simulink library "SDC_decoder_lib"  (Simulink 7.4)
settings: Solver=ode45  StartTime=0.0  StopTime=10.0  RelTol=1e-3
values from neighbouring files (symbols this model uses):
  sPunc_pat = struct( 'Rp16' ,{[1 1 1 1 1 1]' 1 6}, 'Rp14' ,{[1 1 1 1 0 0]' 1 4}, 'Rp310',{[1 1 1 1 0 0 1 1 1 0 0 0 1 1 1 0 0 0]' 3 10}, 'Rp13' ,{[1 1 1 0 0 0]' 1 3}, 'Rp411',{[1 1 1 0 0 0 1 1 1 0 0 0 1 1 1 0 0 0 1 1 0 0 0 0]' 4 11}, 'Rp25',{[1 1 1 0 0 0 1 1 0 0 0]' 2 5}, 'Rp12',{[1 1 0 0 0 0]' 1 2}, 'Rp47' ,{[1 1 0 0 0 0 1 0 1 0 0 0 1 1 0 0 0 0 1 0 0 0 0 0]' 4 7}, 'Rp35' ,{[1 1 0 0 0 0 1 0 0 0 0 0 1 1 0 0 0 0] ...(+501 chars)    [conv_and_puncturing.m]
undefined symbols (not defined in the file or in its folder): sdc
libraries: dspmtrx3 x9, commsequence2 x6, commutil2 x3, commcnvcod2 x3, commblkintrlv2 x3, dspbuff3 x3, commdigbbndam3 x2, SDC_decoder_lib x1
settings Model: Creator=Kevin  LastModifiedBy=Kevin

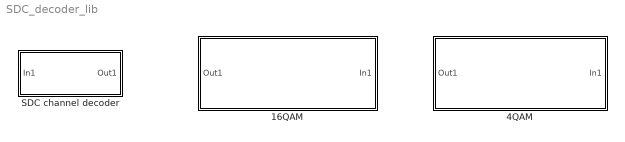
== system SDC_decoder_lib ==
  16QAM : Subsystem
  4QAM : Subsystem
  SDC channel decoder : Subsystem  BlockChoice=16QAM
      settings: TemplateBlock=self  MemberBlocks=16QAM,4QAM

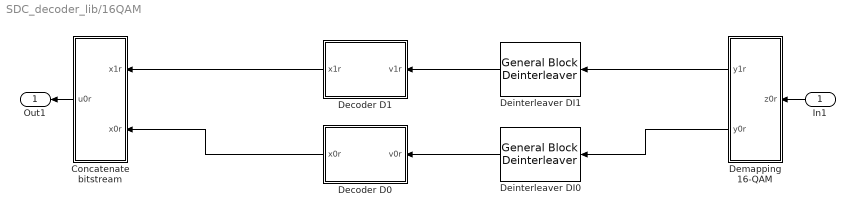
== system SDC_decoder_lib/16QAM ==
  In1 : Inport
  Concatenate bitstream : Subsystem
  Decoder D0 : Subsystem
  Decoder D1 : Subsystem
  Deinterleaver DI0 : commblkintrlv2/General Block Deinterleaver  elements=sdc.interleave_P0
  Deinterleaver DI1 : commblkintrlv2/General Block Deinterleaver  elements=sdc.interleave_P1
  Demapping 16-QAM : Subsystem
  Out1 : Outport
  wires:
  Deinterleaver DI0/1 -> Decoder D0/1(v0r)
  Deinterleaver DI1/1 -> Decoder D1/1(v1r)
  Decoder D0/1(x0r) -> Concatenate bitstream/2(x0r)
  Decoder D1/1(x1r) -> Concatenate bitstream/1(x1r)
  Demapping 16-QAM/2(y0r) -> Deinterleaver DI0/1
  Demapping 16-QAM/1(y1r) -> Deinterleaver DI1/1
  Concatenate bitstream/1(u0r) -> Out1/1
  In1/1 -> Demapping 16-QAM/1(z0r)

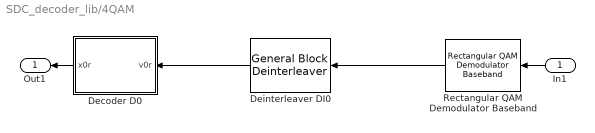
== system SDC_decoder_lib/4QAM ==
  In1 : Inport
  Decoder D0 : Subsystem
  Deinterleaver DI0 : commblkintrlv2/General Block Deinterleaver  elements=sdc.interleave_P0
  Rectangular QAM Demodulator Baseband : commdigbbndam3/Rectangular QAM Demodulator Baseband  DialogController=commDDGCreate  DialogControllerArgs=DataTag4  M=SDC_QAM  PowType=Min. distance between symbols  MinDist=sdc.qam_norm  AvgPow=1  PeakPow=1  Ph=0  Dec=User-defined  Mapping=sdc.qam_map  OutType=Bit  DecType=Hard decision  VarSource=Dialog  Variance=1  outDtype1=Inherit via internal rule  outDtype2=Inherit via internal rule  derotateFactorWordLen=16  denormFactorWordLen=16  prodOutWordLen=32  prodOutRoundingMode=Floor  prodOutOverflowMode=Wrap  sumWordLen=32
  Out1 : Outport
  wires:
  Rectangular QAM Demodulator Baseband/1 -> Deinterleaver DI0/1
  Deinterleaver DI0/1 -> Decoder D0/1(v0r)
  Decoder D0/1(x0r) -> Out1/1
  In1/1 -> Rectangular QAM Demodulator Baseband/1

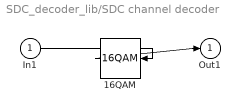
== system SDC_decoder_lib/SDC channel decoder ==
  In1 : Inport
  16QAM : SDC_decoder_lib/16QAM  SystemSampleTime=-1
  Out1 : Outport
  wires:
  In1/1 -> 16QAM/1
  16QAM/1 -> Out1/1

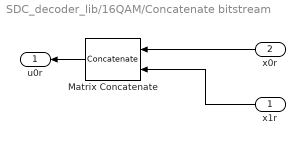
== system SDC_decoder_lib/16QAM/Concatenate bitstream ==
  x1r : Inport
  x0r : Inport  Port=2
  Matrix Concatenate : Concatenate  Mode=Multidimensional array
  u0r : Outport
  wires:
  Matrix Concatenate/1 -> u0r/1
  x0r/1 -> Matrix Concatenate/1
  x1r/1 -> Matrix Concatenate/2

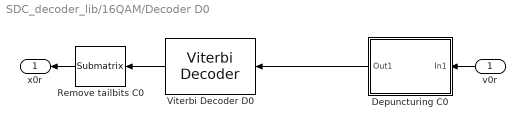
== system SDC_decoder_lib/16QAM/Decoder D0 ==
  v0r : Inport
  Depuncturing C0 : Subsystem
  Remove tailbits C0 : dspmtrx3/Submatrix  RowSpan=Range of rows  RowStartMode=First  RowStartIndex=1  RowEndMode=Offset from last  RowEndIndex=6  ColSpan=All columns  ColStartMode=First  ColStartIndex=1  ColEndMode=Last  ColEndIndex=1
  Viterbi Decoder D0 : commcnvcod2/Viterbi Decoder  DialogController=commDDGCreate  DialogControllerArgs=DataTag0  trellis=conv_poly  isPunctured=off  punctureVector=sPunc_pat(1).Rp13  erasures=off  dectype=Unquantized  runSigValErrCheck=on  nsdecb=3  smWordLength=16  tbdepth=34  opmode=Terminated  reset=off  outDataType=Inherit via internal rule
  x0r : Outport
  wires:
  Remove tailbits C0/1 -> x0r/1
  v0r/1 -> Depuncturing C0/1(In1)
  Depuncturing C0/1(Out1) -> Viterbi Decoder D0/1
  Viterbi Decoder D0/1 -> Remove tailbits C0/1

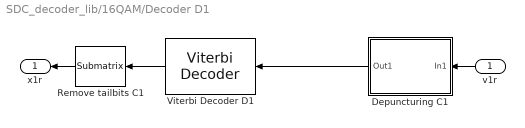
== system SDC_decoder_lib/16QAM/Decoder D1 ==
  v1r : Inport
  Depuncturing C1 : Subsystem
  Remove tailbits C1 : dspmtrx3/Submatrix  RowSpan=Range of rows  RowStartMode=First  RowStartIndex=1  RowEndMode=Offset from last  RowEndIndex=6  ColSpan=All columns  ColStartMode=First  ColStartIndex=1  ColEndMode=Last  ColEndIndex=1
  Viterbi Decoder D1 : commcnvcod2/Viterbi Decoder  DialogController=commDDGCreate  DialogControllerArgs=DataTag1  trellis=conv_poly  isPunctured=off  punctureVector=sPunc_pat(1).Rp23  erasures=off  dectype=Unquantized  runSigValErrCheck=on  nsdecb=3  smWordLength=16  tbdepth=34  opmode=Terminated  reset=off  outDataType=Inherit via internal rule
  x1r : Outport
  wires:
  Remove tailbits C1/1 -> x1r/1
  v1r/1 -> Depuncturing C1/1(In1)
  Depuncturing C1/1(Out1) -> Viterbi Decoder D1/1
  Viterbi Decoder D1/1 -> Remove tailbits C1/1

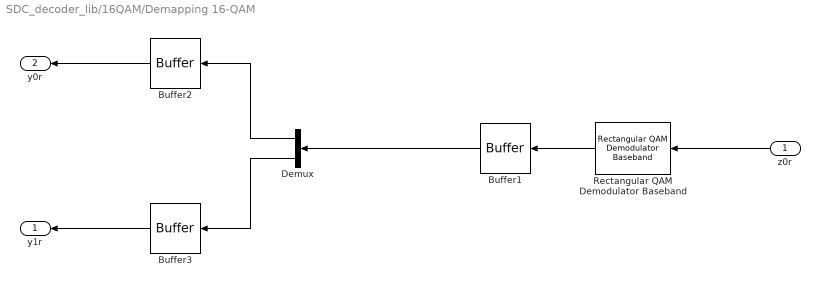
== system SDC_decoder_lib/16QAM/Demapping 16-QAM ==
  z0r : Inport
  Buffer1 : dspbuff3/Buffer  N=2  V=0  ic=0
  Buffer2 : dspbuff3/Buffer  N=2*sdc.NmbQAMcells  V=0  ic=0
  Buffer3 : dspbuff3/Buffer  N=2*sdc.NmbQAMcells  V=0  ic=0
  Demux : Demux  Outputs=2
  Rectangular QAM Demodulator Baseband : commdigbbndam3/Rectangular QAM Demodulator Baseband  DialogController=commDDGCreate  DialogControllerArgs=DataTag2  M=SDC_QAM  PowType=Min. distance between symbols  MinDist=sdc.qam_norm  AvgPow=1  PeakPow=1  Ph=0  Dec=User-defined  Mapping=sdc.qam_map  OutType=Bit  DecType=Hard decision  VarSource=Dialog  Variance=1  outDtype1=Inherit via internal rule  outDtype2=Inherit via internal rule  derotateFactorWordLen=16  denormFactorWordLen=16  prodOutWordLen=32  prodOutRoundingMode=Floor  prodOutOverflowMode=Wrap  sumWordLen=32
  y1r : Outport
  y0r : Outport  Port=2
  wires:
  z0r/1 -> Rectangular QAM Demodulator Baseband/1
  Rectangular QAM Demodulator Baseband/1 -> Buffer1/1
  Demux/2 -> Buffer3/1
  Demux/1 -> Buffer2/1
  Buffer2/1 -> y0r/1
  Buffer3/1 -> y1r/1
  Buffer1/1 -> Demux/1

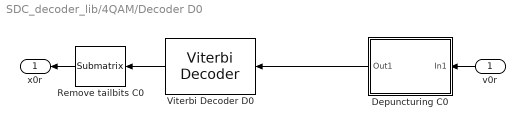
== system SDC_decoder_lib/4QAM/Decoder D0 ==
  v0r : Inport
  Depuncturing C0 : Subsystem
  Remove tailbits C0 : dspmtrx3/Submatrix  RowSpan=Range of rows  RowStartMode=First  RowStartIndex=1  RowEndMode=Offset from last  RowEndIndex=6  ColSpan=All columns  ColStartMode=First  ColStartIndex=1  ColEndMode=Last  ColEndIndex=1
  Viterbi Decoder D0 : commcnvcod2/Viterbi Decoder  DialogController=commDDGCreate  DialogControllerArgs=DataTag3  trellis=conv_poly  isPunctured=off  punctureVector=sPunc_pat(1).Rp13  erasures=off  dectype=Unquantized  runSigValErrCheck=on  nsdecb=3  smWordLength=16  tbdepth=34  opmode=Terminated  reset=off  outDataType=Inherit via internal rule
  x0r : Outport
  wires:
  Remove tailbits C0/1 -> x0r/1
  v0r/1 -> Depuncturing C0/1(In1)
  Depuncturing C0/1(Out1) -> Viterbi Decoder D0/1
  Viterbi Decoder D0/1 -> Remove tailbits C0/1

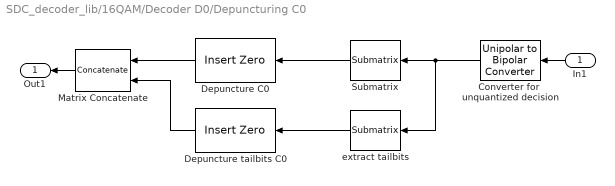
== system SDC_decoder_lib/16QAM/Decoder D0/Depuncturing C0 ==
  In1 : Inport
  Converter for  unquantized decision : commutil2/Unipolar to Bipolar Converter  SystemSampleTime=-1  M=2  polarity=Negative  dataType=Inherit via internal rule
  Depuncture C0 : commsequence2/Insert Zero  insertZeroVector=sdc.punc_pat0
  Depuncture tailbits C0 : commsequence2/Insert Zero  insertZeroVector=sdc.punc_tail0
  Matrix Concatenate : Concatenate  Mode=Multidimensional array
  Submatrix : dspmtrx3/Submatrix  RowSpan=Range of rows  RowStartMode=First  RowStartIndex=1  RowEndMode=Offset from last  RowEndIndex=sdc.ind_tail0  ColSpan=All columns  ColStartMode=First  ColStartIndex=1  ColEndMode=Last  ColEndIndex=1
  extract tailbits : dspmtrx3/Submatrix  RowSpan=Range of rows  RowStartMode=Offset from last  RowStartIndex=sdc.ind_tail0-1  RowEndMode=Last  RowEndIndex=35  ColSpan=All columns  ColStartMode=First  ColStartIndex=1  ColEndMode=Last  ColEndIndex=1
  Out1 : Outport
  wires:
  Matrix Concatenate/1 -> Out1/1
  In1/1 -> Converter for  unquantized decision/1
  Converter for  unquantized decision/1 -> Submatrix/1, extract tailbits/1
  extract tailbits/1 -> Depuncture tailbits C0/1
  Submatrix/1 -> Depuncture C0/1
  Depuncture tailbits C0/1 -> Matrix Concatenate/2
  Depuncture C0/1 -> Matrix Concatenate/1

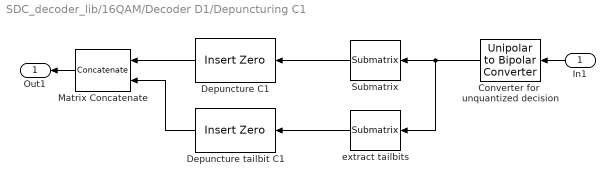
== system SDC_decoder_lib/16QAM/Decoder D1/Depuncturing C1 ==
  In1 : Inport
  Converter for  unquantized decision : commutil2/Unipolar to Bipolar Converter  SystemSampleTime=-1  M=2  polarity=Negative  dataType=Inherit via internal rule
  Depuncture C1 : commsequence2/Insert Zero  insertZeroVector=sdc.punc_pat1
  Depuncture tailbit C1 : commsequence2/Insert Zero  insertZeroVector=sdc.punc_tail1
  Matrix Concatenate : Concatenate  Mode=Multidimensional array
  Submatrix : dspmtrx3/Submatrix  RowSpan=Range of rows  RowStartMode=First  RowStartIndex=1  RowEndMode=Offset from last  RowEndIndex=sdc.ind_tail1  ColSpan=All columns  ColStartMode=First  ColStartIndex=1  ColEndMode=Last  ColEndIndex=1
  extract tailbits : dspmtrx3/Submatrix  RowSpan=Range of rows  RowStartMode=Offset from last  RowStartIndex=sdc.ind_tail1-1  RowEndMode=Last  RowEndIndex=35  ColSpan=All columns  ColStartMode=First  ColStartIndex=1  ColEndMode=Last  ColEndIndex=1
  Out1 : Outport
  wires:
  Matrix Concatenate/1 -> Out1/1
  In1/1 -> Converter for  unquantized decision/1
  Converter for  unquantized decision/1 -> Submatrix/1, extract tailbits/1
  Depuncture tailbit C1/1 -> Matrix Concatenate/2
  extract tailbits/1 -> Depuncture tailbit C1/1
  Depuncture C1/1 -> Matrix Concatenate/1
  Submatrix/1 -> Depuncture C1/1

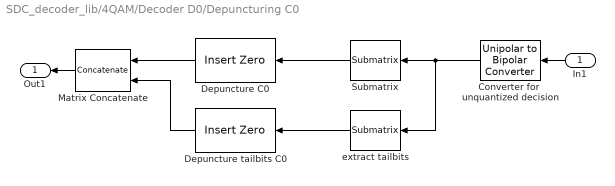
== system SDC_decoder_lib/4QAM/Decoder D0/Depuncturing C0 ==
  In1 : Inport
  Converter for  unquantized decision : commutil2/Unipolar to Bipolar Converter  SystemSampleTime=-1  M=2  polarity=Negative  dataType=Inherit via internal rule
  Depuncture C0 : commsequence2/Insert Zero  insertZeroVector=sdc.punc_pat0
  Depuncture tailbits C0 : commsequence2/Insert Zero  insertZeroVector=sdc.punc_tail0
  Matrix Concatenate : Concatenate  Mode=Multidimensional array
  Submatrix : dspmtrx3/Submatrix  RowSpan=Range of rows  RowStartMode=First  RowStartIndex=1  RowEndMode=Offset from last  RowEndIndex=sdc.ind_tail0  ColSpan=All columns  ColStartMode=First  ColStartIndex=1  ColEndMode=Last  ColEndIndex=1
  extract tailbits : dspmtrx3/Submatrix  RowSpan=Range of rows  RowStartMode=Offset from last  RowStartIndex=sdc.ind_tail0-1  RowEndMode=Last  RowEndIndex=35  ColSpan=All columns  ColStartMode=First  ColStartIndex=1  ColEndMode=Last  ColEndIndex=1
  Out1 : Outport
  wires:
  Matrix Concatenate/1 -> Out1/1
  In1/1 -> Converter for  unquantized decision/1
  Converter for  unquantized decision/1 -> Submatrix/1, extract tailbits/1
  extract tailbits/1 -> Depuncture tailbits C0/1
  Submatrix/1 -> Depuncture C0/1
  Depuncture tailbits C0/1 -> Matrix Concatenate/2
  Depuncture C0/1 -> Matrix Concatenate/1
